simulink model "subsystem_Wheel_speed"  (R2020b)
settings: Solver=VariableStepAuto  StartTime=0.0  StopTime=10.0  RelTol=1e-3
undefined symbols (not defined in the file): I, Kf, PBmax, Rr, TB, v0
settings Model: Creator=lenovo  LastModifiedBy=lenovo

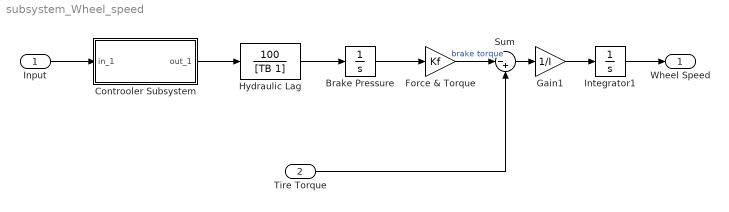
== system subsystem_Wheel_speed ==
  Input : Inport
  Tire Torque : Inport  Port=2
  " Controoler Subsystem" : Subsystem
  Brake Pressure : Integrator  LimitOutput=on  UpperSaturationLimit=PBmax  LowerSaturationLimit=0
  Force & Torque : Gain  Gain=Kf
  Gain1 : Gain  Gain=1/I
  Hydraulic Lag : TransferFcn  Numerator=[100]  Denominator=[TB 1]
  Integrator1 : Integrator  InitialCondition=v0/Rr  LimitOutput=on  UpperSaturationLimit=1000  LowerSaturationLimit=0
  Sum : Sum  Inputs=|-+
  Wheel Speed : Outport
  wires:
  Input/1 -> " Controoler Subsystem"/1(in_1)
  " Controoler Subsystem"/1(out_1) -> Hydraulic Lag/1
  Hydraulic Lag/1 -> Brake Pressure/1
  Brake Pressure/1 -> Force & Torque/1
  Force & Torque/1 -> Sum/1  "brake torque"
  Sum/1 -> Gain1/1
  Integrator1/1 -> Wheel Speed/1
  Gain1/1 -> Integrator1/1
  Tire Torque/1 -> Sum/2

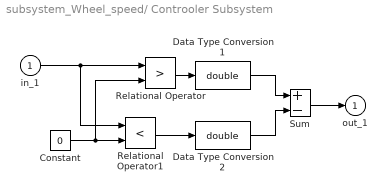
== system subsystem_Wheel_speed/ Controoler Subsystem ==
  in_1 : Inport
  Constant : Constant  Value=0
  Data Type Conversion1 : DataTypeConversion  OutDataTypeStr=double  SaturateOnIntegerOverflow=on  RndMeth=Zero
  Data Type Conversion2 : DataTypeConversion  OutDataTypeStr=double  SaturateOnIntegerOverflow=on  RndMeth=Zero
  Relational Operator : RelationalOperator  Operator=>  OutDataTypeStr=boolean  RndMeth=Nearest  InputSameDT=on
  Relational Operator1 : RelationalOperator  Operator=<  OutDataTypeStr=boolean  RndMeth=Nearest  InputSameDT=on
  Sum : Sum  Inputs=+-  InputSameDT=on  SaturateOnIntegerOverflow=on  OutDataTypeStr=Inherit: Same as first input
  out_1 : Outport  InitialOutput=0  VectorParamsAs1DForOutWhenUnconnected=off
  wires:
  in_1/1 -> Relational Operator/1, Relational Operator1/1
  Constant/1 -> Relational Operator1/2, Relational Operator/2
  Relational Operator1/1 -> Data Type Conversion2/1
  Relational Operator/1 -> Data Type Conversion1/1
  Sum/1 -> out_1/1
  Data Type Conversion1/1 -> Sum/1
  Data Type Conversion2/1 -> Sum/2
